simulink model "simulink_model"  (R2025b)
settings: Solver=VariableStepAuto  StartTime=0.0  StopTime=10.0  RelTol=1e-3
libraries: fuzblock x1
settings Model: Creator=nehor  LastModifiedBy=nehor

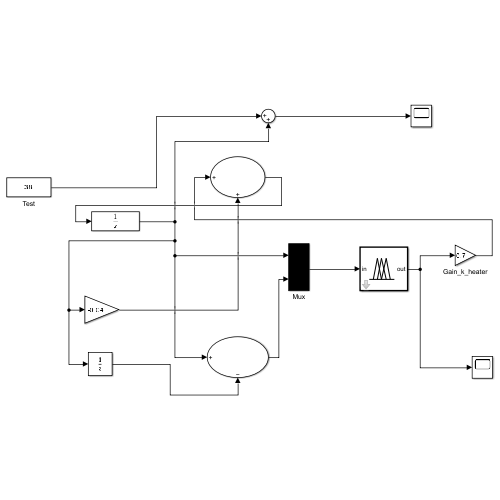
[thumbnail: Simulink's stored preview of the top-level diagram]
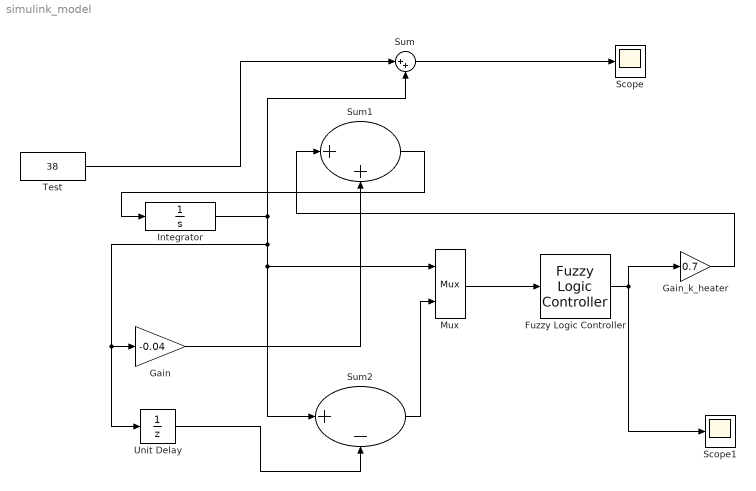
== system simulink_model ==
  Fuzzy Logic Controller : fuzblock/Fuzzy Logic  Controller  FIS='sugenotype1.fis'  OutputSampleNumber=101  DataType=double  UseLookupTable=off  NumBreakpoints=10  FuzzifiedInputs=off  RuleFiringStrengths=off  RuleOutputs=off  AggregatedOutputs=off  SimulateUsing=Interpreted execution  OutOfRangeInputValueMessage=warning  NoRuleFiredMessage=warning  EmptyOutputFuzzySetMessage=warning
  Gain : Gain  Gain=-0.04
  Gain_k_heater : Gain  Gain=0.7
  Integrator : Integrator
  Mux : Mux  Inputs=2
  Scope : Scope
  Scope1 : Scope
  Sum : Sum  Inputs=|++
  Sum1 : Sum  Inputs=|++
  Sum2 : Sum  Inputs=|+-
  Test : Constant  Value=38
  Unit Delay : UnitDelay  SampleTime=-1  HasFrameUpgradeWarning=on
  wires:
  Fuzzy Logic Controller/1 -> Gain_k_heater/1, Scope1/1
  Sum/1 -> Scope/1
  Mux/1 -> Fuzzy Logic Controller/1
  Test/1 -> Sum/1
  Sum1/1 -> Integrator/1
  Integrator/1 -> Sum2/1, Mux/1, Unit Delay/1, Gain/1, Sum/2
  Gain/1 -> Sum1/2
  Unit Delay/1 -> Sum2/2
  Sum2/1 -> Mux/2
  Gain_k_heater/1 -> Sum1/1
